simulink subsystem "rss_CtlBrdVltgHiLvl1Dia"  (R2023a)
settings: Solver=VariableStepAuto  StartTime=0.0  StopTime=10.0  RelTol=1e-3
undefined symbols (not defined in the file): Cdbl_uCtlBrdVltgMaxVal, ENM_TYPE_FALT, Gu16_ctCtlBrdVltgHiLvl1ConfCnt_C, Gu16_ctCtlBrdVltgHiLvl1RcvyCnt_C, Gu16_uCtlBrdVltgHiLvl1ConfTrs_C, Gu16_uCtlBrdVltgHiLvl1RcvyTrs_C
libraries: vhit_control_library x1, lib_fault_definiteness x1
settings Model: Creator=xiaoqiang.yuan  LastModifiedBy=xiaoqiang.yuan

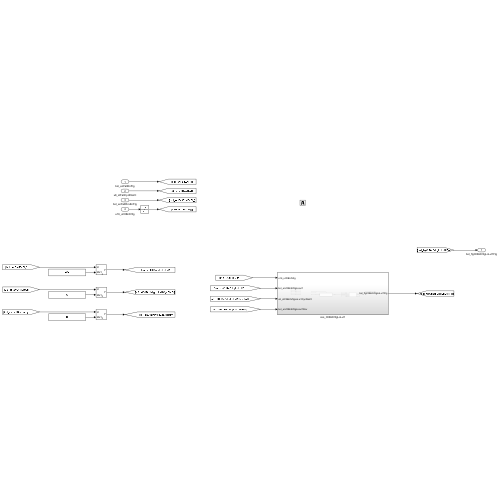
[thumbnail: Simulink's stored preview of the top-level diagram]
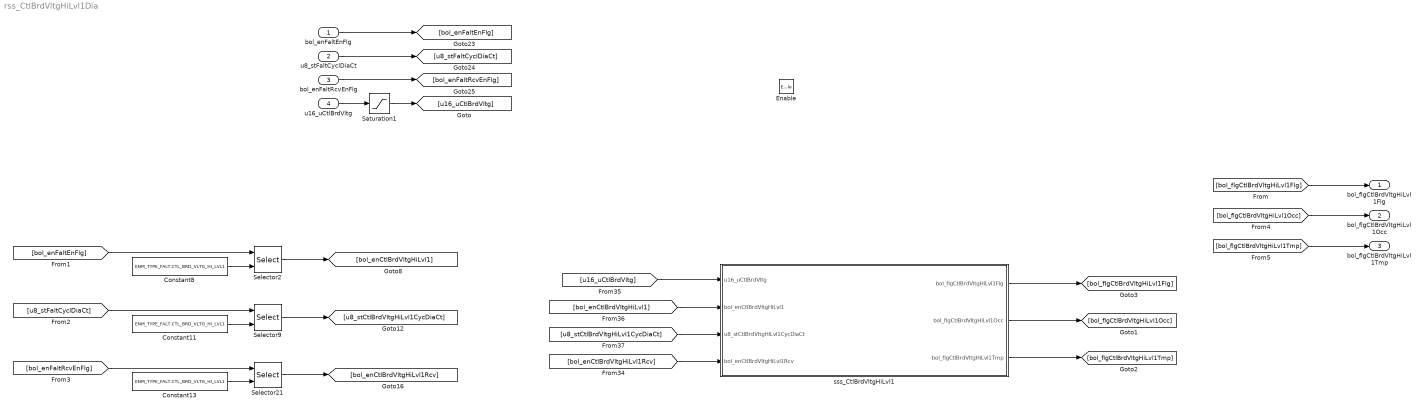
== system rss_CtlBrdVltgHiLvl1Dia ==
  bol_enFaltEnFlg : Inport  OutDataTypeStr=boolean
  u8_stFaltCyclDiaCt : Inport  Port=2  OutDataTypeStr=uint8
  bol_enFaltRcvEnFlg : Inport  Port=3  OutDataTypeStr=boolean
  u16_uCtlBrdVltg : Inport  Port=4  OutDataTypeStr=dt_Standardize_u16p15b0
  Enable : EnablePort
  Constant11 : Constant  Value=ENM_TYPE_FALT.CTL_BRD_VLTG_HI_LVL1
  Constant13 : Constant  Value=ENM_TYPE_FALT.CTL_BRD_VLTG_HI_LVL1
  Constant8 : Constant  Value=ENM_TYPE_FALT.CTL_BRD_VLTG_HI_LVL1
  Saturation1 : Saturate  UpperLimit=Cdbl_uCtlBrdVltgMaxVal  LowerLimit=0
  Selector2 : Selector  IndexMode=Zero-based  InputPortWidth=Cdbl_numFaltDiaNum  IndexOptions=Index vector (port)  Indices=[1 3]  OutputSizes=1
  Selector21 : Selector  IndexMode=Zero-based  InputPortWidth=Cdbl_numFaltDiaNum  IndexOptions=Index vector (port)  Indices=[1 3]  OutputSizes=1
  Selector9 : Selector  IndexMode=Zero-based  InputPortWidth=Cdbl_numFaltDiaNum  IndexOptions=Index vector (port)  Indices=[1 3]  OutputSizes=1
  sss_CtlBrdVltgHiLvl1 : Subsystem
  bol_flgCtlBrdVltgHiLvl1Flg : Outport  OutDataTypeStr=boolean
  bol_flgCtlBrdVltgHiLvl1Occ : Outport  Port=2  OutDataTypeStr=boolean
  bol_flgCtlBrdVltgHiLvl1Tmp : Outport  Port=3  OutDataTypeStr=boolean
  wires:
  [bol_flgCtlBrdVltgHiLvl1Flg] -> bol_flgCtlBrdVltgHiLvl1Flg/1
  [u16_uCtlBrdVltg] -> sss_CtlBrdVltgHiLvl1/1(u16_uCtlBrdVltg)
  [u8_stCtlBrdVltgHiLvl1CycDiaCt] -> sss_CtlBrdVltgHiLvl1/3(u8_stCtlBrdVltgHiLvl1CycDiaCt)
  [bol_enCtlBrdVltgHiLvl1] -> sss_CtlBrdVltgHiLvl1/2(bol_enCtlBrdVltgHiLvl1)
  sss_CtlBrdVltgHiLvl1/1(bol_flgCtlBrdVltgHiLvl1Flg) -> [bol_flgCtlBrdVltgHiLvl1Flg]
  [bol_enCtlBrdVltgHiLvl1Rcv] -> sss_CtlBrdVltgHiLvl1/4(bol_enCtlBrdVltgHiLvl1Rcv)
  u16_uCtlBrdVltg/1 -> Saturation1/1
  u8_stFaltCyclDiaCt/1 -> [u8_stFaltCyclDiaCt]
  bol_enFaltRcvEnFlg/1 -> [bol_enFaltRcvEnFlg]
  bol_enFaltEnFlg/1 -> [bol_enFaltEnFlg]
  [u8_stFaltCyclDiaCt] -> Selector9/1
  [bol_enFaltRcvEnFlg] -> Selector21/1
  [bol_enFaltEnFlg] -> Selector2/1
  Selector21/1 -> [bol_enCtlBrdVltgHiLvl1Rcv]
  Selector9/1 -> [u8_stCtlBrdVltgHiLvl1CycDiaCt]
  Selector2/1 -> [bol_enCtlBrdVltgHiLvl1]
  Constant11/1 -> Selector9/2
  Constant13/1 -> Selector21/2
  Constant8/1 -> Selector2/2
  Saturation1/1 -> [u16_uCtlBrdVltg]
  sss_CtlBrdVltgHiLvl1/2(bol_flgCtlBrdVltgHiLvl1Occ) -> [bol_flgCtlBrdVltgHiLvl1Occ]
  [bol_flgCtlBrdVltgHiLvl1Occ] -> bol_flgCtlBrdVltgHiLvl1Occ/1
  [bol_flgCtlBrdVltgHiLvl1Tmp] -> bol_flgCtlBrdVltgHiLvl1Tmp/1
  sss_CtlBrdVltgHiLvl1/3(bol_flgCtlBrdVltgHiLvl1Tmp) -> [bol_flgCtlBrdVltgHiLvl1Tmp]

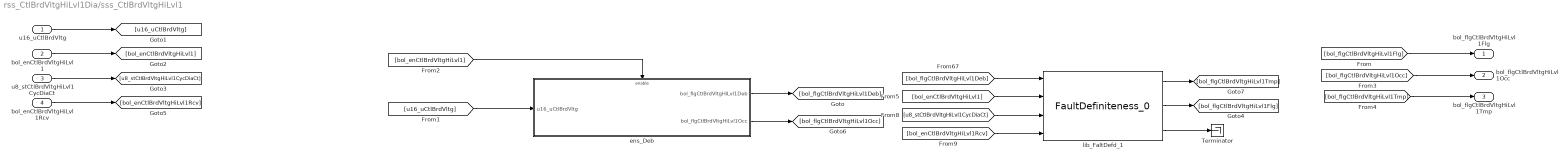
== system rss_CtlBrdVltgHiLvl1Dia/sss_CtlBrdVltgHiLvl1 ==
  u16_uCtlBrdVltg : Inport
  bol_enCtlBrdVltgHiLvl1 : Inport  Port=2
  u8_stCtlBrdVltgHiLvl1CycDiaCt : Inport  Port=3
  bol_enCtlBrdVltgHiLvl1Rcv : Inport  Port=4
  Terminator : Terminator
  ens_Deb : Subsystem
  lib_FaltDefd_1 : lib_fault_definiteness/FaultDefiniteness_0  lb_FaltWaitRecvCnt=Gu16_ctCtlBrdVltgHiLvl1ConfCnt_C
  bol_flgCtlBrdVltgHiLvl1Flg : Outport
  bol_flgCtlBrdVltgHiLvl1Occ : Outport  Port=2
  bol_flgCtlBrdVltgHiLvl1Tmp : Outport  Port=3
  wires:
  [bol_flgCtlBrdVltgHiLvl1Tmp] -> bol_flgCtlBrdVltgHiLvl1Tmp/1
  [bol_flgCtlBrdVltgHiLvl1Occ] -> bol_flgCtlBrdVltgHiLvl1Occ/1
  ens_Deb/2(bol_flgCtlBrdVltgHiLvl1Occ) -> [bol_flgCtlBrdVltgHiLvl1Occ]
  lib_FaltDefd_1/1 -> [bol_flgCtlBrdVltgHiLvl1Tmp]
  lib_FaltDefd_1/2 -> [bol_flgCtlBrdVltgHiLvl1Flg]
  lib_FaltDefd_1/3 -> Terminator/1
  [bol_enCtlBrdVltgHiLvl1] -> ens_Deb/Enable
  [u16_uCtlBrdVltg] -> ens_Deb/1(u16_uCtlBrdVltg)
  ens_Deb/1(bol_flgCtlBrdVltgHiLvl1Deb) -> [bol_flgCtlBrdVltgHiLvl1Deb]
  bol_enCtlBrdVltgHiLvl1Rcv/1 -> [bol_enCtlBrdVltgHiLvl1Rcv]
  u8_stCtlBrdVltgHiLvl1CycDiaCt/1 -> [u8_stCtlBrdVltgHiLvl1CycDiaCt]
  bol_enCtlBrdVltgHiLvl1/1 -> [bol_enCtlBrdVltgHiLvl1]
  [bol_flgCtlBrdVltgHiLvl1Flg] -> bol_flgCtlBrdVltgHiLvl1Flg/1
  u16_uCtlBrdVltg/1 -> [u16_uCtlBrdVltg]
  [bol_enCtlBrdVltgHiLvl1Rcv] -> lib_FaltDefd_1/4
  [u8_stCtlBrdVltgHiLvl1CycDiaCt] -> lib_FaltDefd_1/3
  [bol_enCtlBrdVltgHiLvl1] -> lib_FaltDefd_1/2
  [bol_flgCtlBrdVltgHiLvl1Deb] -> lib_FaltDefd_1/1

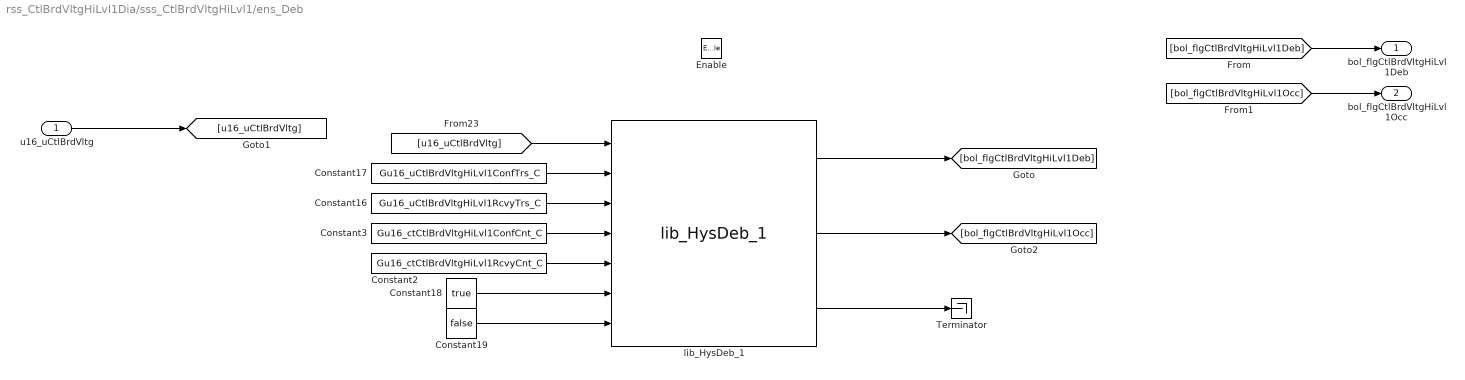
== system rss_CtlBrdVltgHiLvl1Dia/sss_CtlBrdVltgHiLvl1/ens_Deb ==
  u16_uCtlBrdVltg : Inport
  Enable : EnablePort
  Constant16 : Constant  Value=Gu16_uCtlBrdVltgHiLvl1RcvyTrs_C
  Constant17 : Constant  Value=Gu16_uCtlBrdVltgHiLvl1ConfTrs_C
  Constant18 : Constant  Value=true  OutDataTypeStr=boolean
  Constant19 : Constant  Value=false  OutDataTypeStr=boolean
  Constant2 : Constant  Value=Gu16_ctCtlBrdVltgHiLvl1RcvyCnt_C
  Constant3 : Constant  Value=Gu16_ctCtlBrdVltgHiLvl1ConfCnt_C
  Terminator : Terminator
  lib_HysDeb_1 : vhit_control_library/lib_HysDeb_1  lb_parInitOutp=0
  bol_flgCtlBrdVltgHiLvl1Deb : Outport
  bol_flgCtlBrdVltgHiLvl1Occ : Outport  Port=2
  wires:
  Constant2/1 -> lib_HysDeb_1/5
  Constant3/1 -> lib_HysDeb_1/4
  Constant16/1 -> lib_HysDeb_1/3
  Constant17/1 -> lib_HysDeb_1/2
  [bol_flgCtlBrdVltgHiLvl1Occ] -> bol_flgCtlBrdVltgHiLvl1Occ/1
  lib_HysDeb_1/3 -> Terminator/1
  lib_HysDeb_1/2 -> [bol_flgCtlBrdVltgHiLvl1Occ]
  Constant19/1 -> lib_HysDeb_1/7
  Constant18/1 -> lib_HysDeb_1/6
  [u16_uCtlBrdVltg] -> lib_HysDeb_1/1
  u16_uCtlBrdVltg/1 -> [u16_uCtlBrdVltg]
  [bol_flgCtlBrdVltgHiLvl1Deb] -> bol_flgCtlBrdVltgHiLvl1Deb/1
  lib_HysDeb_1/1 -> [bol_flgCtlBrdVltgHiLvl1Deb]
